simulink model "MPC_block"  (R2021a)
settings: Solver=FixedStepAuto  StartTime=0.0  StopTime=10  FixedStep=0.03  RelTol=1e-3
libraries: mpclib x1
settings Model: Creator=francois  LastModifiedBy=esl
settings SolverCC: AlgebraicLoopSolver=TrustRegion
settings DataIOCC: SaveOutput=off  SaveTime=off
settings DebuggingCC: SFMachineParentedDataDiag=warning
settings RTWCC: Description=Create Visual C/C++ Solution File for Simulink Coder  TemplateMakefile=RTW.MSVCBuild

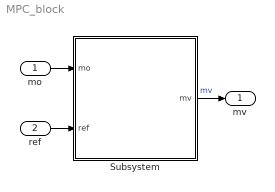
== system MPC_block ==
  mo : Inport  OutDataTypeStr=double  PortDimensions=60  SampleTime=[0.029999999999999999,0]
  ref : Inport  Port=2  OutDataTypeStr=double  PortDimensions=60  SampleTime=[0.029999999999999999,0]
  Subsystem : Subsystem
  mv : Outport  OutDataTypeStr=double  PortDimensions=3  SampleTime=[0.029999999999999999,0]
  wires:
  mo/1 -> Subsystem/1(mo)
  Subsystem/1(mv) -> mv/1  "mv"
  ref/1 -> Subsystem/2(ref)

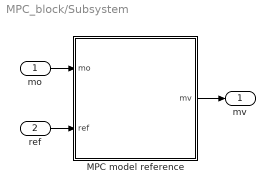
== system MPC_block/Subsystem ==
  mo : Inport
  ref : Inport  Port=2
  MPC model reference : Subsystem  TreatAsAtomicUnit=on
  mv : Outport
  wires:
  mo/1 -> MPC model reference/1(mo)
  ref/1 -> MPC model reference/2(ref)
  MPC model reference/1(mv) -> mv/1

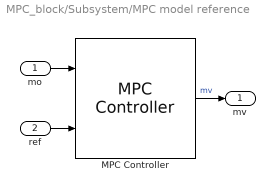
== system MPC_block/Subsystem/MPC model reference ==
  mo : Inport
  ref : Inport  Port=2
  MPC Controller : mpclib/MPC Controller  SCDEnableBlockLinearizationSpecification=on  mpcobj=mpc_vel  is_multiple=0  enable_value=0  return_u0=off  updateMPCinCallerWorkspace=on  md_inport=off  mv_inport=off  uref_inport=off  return_cost=off  return_mvseq=off  return_qpstatus=off  return_xseq=off  return_state=off  return_ovseq=off  state_inport=off  umin_inport=off  umax_inport=off  ymin_inport=off  ymax_inport=off  cc_inport=off  ywt_inport=off  uwt_inport=off  duwt_inport=off  rhoeps_inport=off  pm_inport=off  MaximumP=10  HorizonChoice=FixedHorizon  n_ts=0.03  n_p=200  n_mv=3  n_md=0  n_ud=0  n_mo=60  n_uo=0  BlockDataType=double  SampleTimeInherited=off  switch_inport=off
  mv : Outport
  wires:
  mo/1 -> MPC Controller/1
  MPC Controller/1 -> mv/1  "mv"
  ref/1 -> MPC Controller/2
